simulink model "pos_traj"  (R2017b)
settings: Solver=VariableStepAuto  StartTime=0.0  StopTime=10  RelTol=1e-3
libraries: powerlib_meascontrol x5, mylibrary x2
settings Model: Creator=Kamran  LastModifiedBy=Kamran

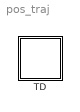
== system pos_traj ==
  TD : Subsystem  mask{h=1e-3, jm=3, am=2, vm=1}

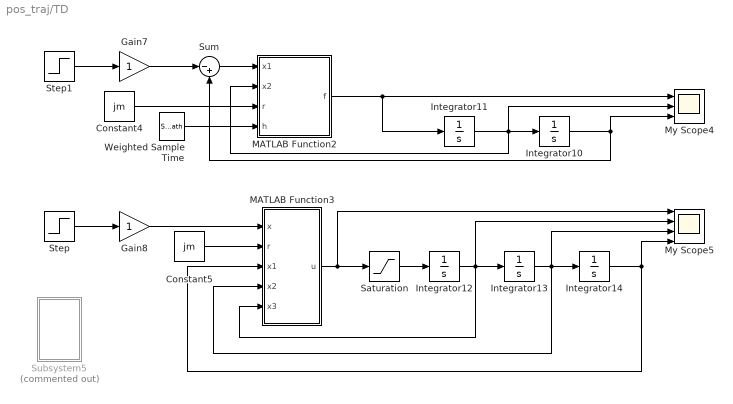
== system pos_traj/TD ==
  Constant4 : Constant  Value=jm
  Constant5 : Constant  Value=jm
  Gain7 : Gain
  Gain8 : Gain
  Integrator10 : Integrator  InitialCondition=0.5  UpperSaturationLimit=vm  LowerSaturationLimit=-vm
  Integrator11 : Integrator  InitialCondition=0.5  LimitOutput=on  UpperSaturationLimit=am  LowerSaturationLimit=-am
  Integrator12 : Integrator  LimitOutput=on  UpperSaturationLimit=sat  LowerSaturationLimit=-sat  ZeroCross=off  mask{sat=am}
  Integrator13 : Integrator  LimitOutput=on  UpperSaturationLimit=sat  LowerSaturationLimit=-sat  ZeroCross=off  mask{sat=vm}
  Integrator14 : Integrator  ZeroCross=off
  MATLAB Function2 : MATLAB Function  TreatAsAtomicUnit=on
  MATLAB Function3 : MATLAB Function  TreatAsAtomicUnit=on
  My Scope4 : Scope  NumInputPorts=3
  My Scope5 : Scope  NumInputPorts=4
  Saturation : Saturate  UpperLimit=sat  LowerLimit=-sat  ZeroCross=off  mask{sat=jm}
  Step : Step  SampleTime=h
  Step1 : Step  Time=0  SampleTime=h
  Subsystem5 : Subsystem  Commented=on
  Sum : Sum  Inputs=|-+
  Weighted Sample Time : SampleTimeMath  TsampMathOp=Ts Only
  wires:
  Saturation/1 -> Integrator12/1
  Integrator12/1 -> My Scope5/2, MATLAB Function3/5(x3), Integrator13/1
  Integrator13/1 -> My Scope5/3, MATLAB Function3/4(x2), Integrator14/1
  Step/1 -> Gain8/1
  Gain8/1 -> MATLAB Function3/1(x)
  MATLAB Function3/1(u) -> Saturation/1, My Scope5/1
  Constant5/1 -> MATLAB Function3/2(r)
  Integrator14/1 -> My Scope5/4, MATLAB Function3/3(x1)
  Integrator10/1 -> Sum/2, My Scope4/3
  Constant4/1 -> MATLAB Function2/3(r)
  Step1/1 -> Gain7/1
  Integrator11/1 -> MATLAB Function2/2(x2), My Scope4/2, Integrator10/1
  Gain7/1 -> Sum/1
  MATLAB Function2/1(f) -> My Scope4/1, Integrator11/1
  Sum/1 -> MATLAB Function2/1(x1)
  Weighted Sample Time/1 -> MATLAB Function2/4(h)

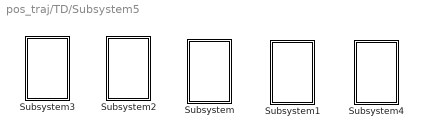
== system pos_traj/TD/Subsystem5 ==
  Subsystem : Subsystem
  Subsystem1 : Subsystem
  Subsystem2 : Subsystem
  Subsystem3 : Subsystem
  Subsystem4 : Subsystem

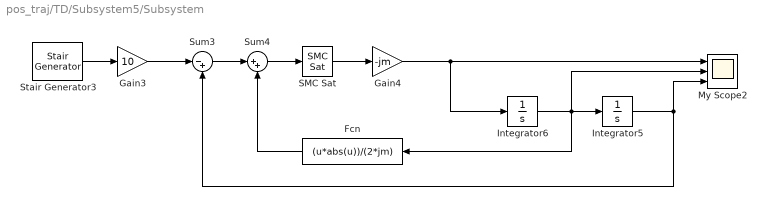
== system pos_traj/TD/Subsystem5/Subsystem ==
  Fcn : Fcn  Expr=(u*abs(u))/(2*jm)
  Gain3 : Gain  Gain=10
  Gain4 : Gain  Gain=-jm
  Integrator5 : Integrator  UpperSaturationLimit=vm  LowerSaturationLimit=-vm
  Integrator6 : Integrator  LimitOutput=on  UpperSaturationLimit=am  LowerSaturationLimit=-am
  My Scope2 : Scope  NumInputPorts=3
  SMC Sat : mylibrary/SMC Sat  psi=eps
      settings: SourceProductName=My Library
  Stair Generator3 : powerlib_meascontrol/Pulse & Signal Generators/Stair Generator  t=[0, 2, 15, 25]  e=[0, 1, 0.1, 0]  Ts=h
      settings: SourceProductName=Simscape Power Systems
  Sum3 : Sum  Inputs=|-+
  Sum4 : Sum  Inputs=|++
  wires:
  Integrator5/1 -> Sum3/2, My Scope2/3
  Sum4/1 -> SMC Sat/1
  Stair Generator3/1 -> Gain3/1
  Gain3/1 -> Sum3/1
  Sum3/1 -> Sum4/1
  Integrator6/1 -> Fcn/1, Integrator5/1, My Scope2/2
  Fcn/1 -> Sum4/2
  Gain4/1 -> Integrator6/1, My Scope2/1
  SMC Sat/1 -> Gain4/1

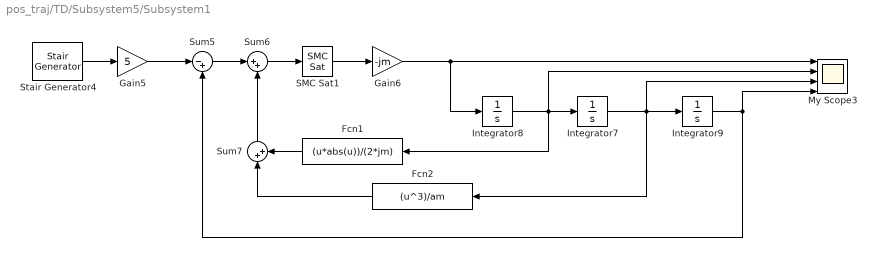
== system pos_traj/TD/Subsystem5/Subsystem1 ==
  Fcn1 : Fcn  Expr=(u*abs(u))/(2*jm)
  Fcn2 : Fcn  Expr=(u^3)/am
  Gain5 : Gain  Gain=5
  Gain6 : Gain  Gain=-jm
  Integrator7 : Integrator  LimitOutput=on  UpperSaturationLimit=vm  LowerSaturationLimit=-vm
  Integrator8 : Integrator  LimitOutput=on  UpperSaturationLimit=am  LowerSaturationLimit=-am
  Integrator9 : Integrator
  My Scope3 : Scope  NumInputPorts=4
  SMC Sat1 : mylibrary/SMC Sat  psi=eps
      settings: SourceProductName=My Library
  Stair Generator4 : powerlib_meascontrol/Pulse & Signal Generators/Stair Generator  t=[0, 2, 15, 25]  e=[0, 1, 0.1, 0]  Ts=h
      settings: SourceProductName=Simscape Power Systems
  Sum5 : Sum  Inputs=|-+
  Sum6 : Sum  Inputs=|++
  Sum7 : Sum  Inputs=|++
  wires:
  Gain6/1 -> My Scope3/1, Integrator8/1
  SMC Sat1/1 -> Gain6/1
  Fcn1/1 -> Sum7/2
  Fcn2/1 -> Sum7/1
  Integrator7/1 -> Fcn2/1, Integrator9/1, My Scope3/3
  Stair Generator4/1 -> Gain5/1
  Sum5/1 -> Sum6/1
  Integrator8/1 -> My Scope3/2, Integrator7/1, Fcn1/1
  Sum6/1 -> SMC Sat1/1
  Integrator9/1 -> Sum5/2, My Scope3/4
  Sum7/1 -> Sum6/2
  Gain5/1 -> Sum5/1

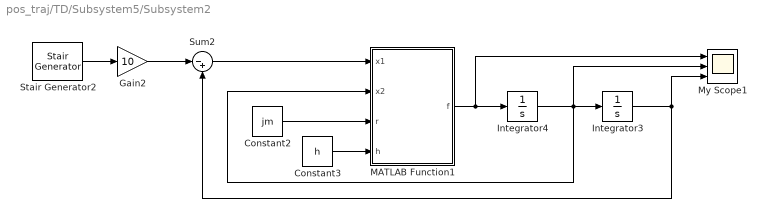
== system pos_traj/TD/Subsystem5/Subsystem2 ==
  Constant2 : Constant  Value=jm
  Constant3 : Constant  Value=h
  Gain2 : Gain  Gain=10
  Integrator3 : Integrator  UpperSaturationLimit=vm  LowerSaturationLimit=-vm
  Integrator4 : Integrator  LimitOutput=on  UpperSaturationLimit=am  LowerSaturationLimit=-am
  MATLAB Function1 : MATLAB Function  TreatAsAtomicUnit=on
  My Scope1 : Scope  NumInputPorts=3
  Stair Generator2 : powerlib_meascontrol/Pulse & Signal Generators/Stair Generator  t=[0, 2, 15, 25]  e=[0, 1, 0.1, 0]  Ts=h
      settings: SourceProductName=Simscape Power Systems
  Sum2 : Sum  Inputs=|-+
  wires:
  Constant3/1 -> MATLAB Function1/4(h)
  Integrator4/1 -> My Scope1/2, MATLAB Function1/2(x2), Integrator3/1
  Sum2/1 -> MATLAB Function1/1(x1)
  Constant2/1 -> MATLAB Function1/3(r)
  Gain2/1 -> Sum2/1
  Integrator3/1 -> My Scope1/3, Sum2/2
  Stair Generator2/1 -> Gain2/1
  MATLAB Function1/1(f) -> My Scope1/1, Integrator4/1

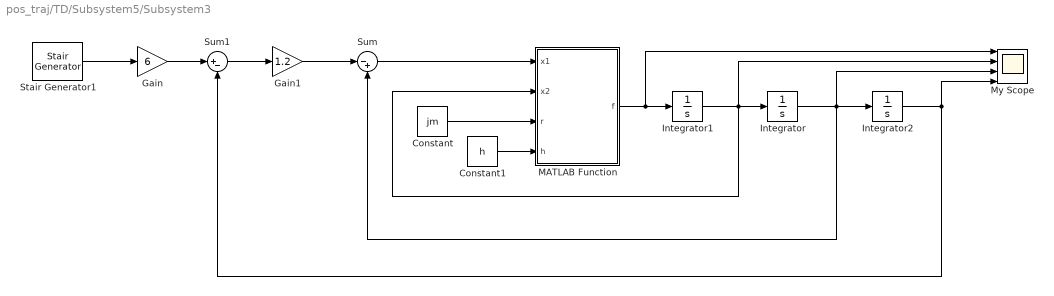
== system pos_traj/TD/Subsystem5/Subsystem3 ==
  Constant : Constant  Value=jm
  Constant1 : Constant  Value=h
  Gain : Gain  Gain=6
  Gain1 : Gain  Gain=1.2
  Integrator : Integrator  LimitOutput=on  UpperSaturationLimit=vm  LowerSaturationLimit=-vm
  Integrator1 : Integrator  LimitOutput=on  UpperSaturationLimit=am  LowerSaturationLimit=-am
  Integrator2 : Integrator
  MATLAB Function : MATLAB Function  TreatAsAtomicUnit=on
  My Scope : Scope  NumInputPorts=4
  Stair Generator1 : powerlib_meascontrol/Pulse & Signal Generators/Stair Generator  t=[0, 2, 15, 25]  e=[0, 1, 0.1, 0]  Ts=h
      settings: SourceProductName=Simscape Power Systems
  Sum : Sum  Inputs=|-+
  Sum1 : Sum  Inputs=|+-
  wires:
  Integrator/1 -> My Scope/3, Sum/2, Integrator2/1
  Constant1/1 -> MATLAB Function/4(h)
  Sum/1 -> MATLAB Function/1(x1)
  Integrator1/1 -> Integrator/1, My Scope/2, MATLAB Function/2(x2)
  Gain1/1 -> Sum/1
  Constant/1 -> MATLAB Function/3(r)
  Gain/1 -> Sum1/1
  Sum1/1 -> Gain1/1
  Stair Generator1/1 -> Gain/1
  Integrator2/1 -> Sum1/2, My Scope/4
  MATLAB Function/1(f) -> My Scope/1, Integrator1/1

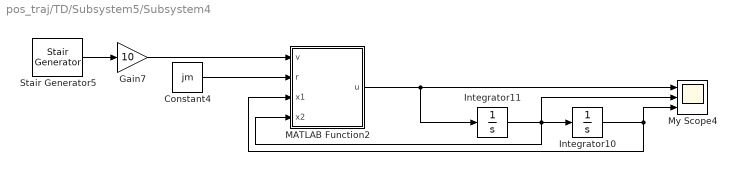
== system pos_traj/TD/Subsystem5/Subsystem4 ==
  Constant4 : Constant  Value=jm
  Gain7 : Gain  Gain=10
  Integrator10 : Integrator  UpperSaturationLimit=vm  LowerSaturationLimit=-vm
  Integrator11 : Integrator  LimitOutput=on  UpperSaturationLimit=am  LowerSaturationLimit=-am
  MATLAB Function2 : MATLAB Function  TreatAsAtomicUnit=on
  My Scope4 : Scope  NumInputPorts=3
  Stair Generator5 : powerlib_meascontrol/Pulse & Signal Generators/Stair Generator  t=[0, 2, 15, 25]  e=[0, 1, 0.1, 0]  Ts=h
      settings: SourceProductName=Simscape Power Systems
  wires:
  Gain7/1 -> MATLAB Function2/1(v)
  MATLAB Function2/1(u) -> My Scope4/1, Integrator11/1
  Integrator11/1 -> MATLAB Function2/4(x2), My Scope4/2, Integrator10/1
  Integrator10/1 -> MATLAB Function2/3(x1), My Scope4/3
  Stair Generator5/1 -> Gain7/1
  Constant4/1 -> MATLAB Function2/2(r)

== matlab function pos_traj/TD/Subsystem5/Subsystem2/MATLAB Function1 ==
  data: x1 input; f output; x2 input; r input; h input
function f = fhan(x1, x2, r, h)

d = r * h^2;
a0 = h * x2;
y = x1 + a0;
a1 = sqrt(d * (d + 8 * abs(y)));
a2 = a0 + sign(y) * (a1 - d) / 2;
sy = (sign(y + d) - sign(y - d)) / 2;
a = (a0 + y - a2) * sy + a2;
sa = (sign(a + d) - sign(a - d)) / 2;
f = -r * (a / d - sign(a)) * sa - r * sign(a);

end

== matlab function pos_traj/TD/Subsystem5/Subsystem4/MATLAB Function2 ==
  data: v input; u output; r input; x1 input; x2 input
function u = fcn(v, r, x1, x2)
    e = v - x1;
    u = r * sat(e - x2 * abs(x2) / (2 * r));
end

function y = sat(s)
    psi = eps;
    if (abs(s) > psi)
        y = sign(s);
    else
        y = s / psi;
    end
end

== matlab function pos_traj/TD/MATLAB Function3 ==
  data: x input; u output; r input; x1 input; x2 input; x3 input
function u  = fcn(x, r, x1, x2, x3)
    s = x1;
    v = x2;
    a = x3;
%     z = v + 0.5 * a * abs(a) / r;
    z = v - a^2/(2*r) * -sat(a);
%     z = s + a^3/(3*r^2) - (a*v)/r * dir(s, v, a);
    u = r * sat(x - z);
end

function d = dir(s, v, a)
    d = 1;
end

function y = sat(s)
    psi = eps;
    if (abs(s) > psi)
        y = sign(s);
    else
        y = s / psi;
    end
end

== matlab function pos_traj/TD/MATLAB Function2 ==
  data: x1 input; x2 input; r input; h input; f output
function f = fhan(x1, x2, r, h)

    d = r * h^2;
    a0 = h * x2;
    y = x1 + a0;
    a1 = sqrt(d * (d + 8 * abs(y)));
    a2 = a0 + sign(y) * (a1 - d) / 2;
    sy = (sign(y + d) - sign(y - d)) / 2;
    a = (a0 + y - a2) * sy + a2;
    sa = (sign(a + d) - sign(a - d)) / 2;
    f = -r * (a / d - sign(a)) * sa - r * sign(a);

end

== matlab function pos_traj/TD/Subsystem5/Subsystem3/MATLAB Function ==
  data: x1 input; f output; x2 input; r input; h input
function f = fhan(x1, x2, r, h)

d = r * h^2;
a0 = h * x2;
y = x1 + a0;
a1 = sqrt(d * (d + 8 * abs(y)));
a2 = a0 + sign(y) * (a1 - d) / 2;
sy = (sign(y + d) - sign(y - d)) / 2;
a = (a0 + y - a2) * sy + a2;
sa = (sign(a + d) - sign(a - d)) / 2;
f = -r * (a / d - sign(a)) * sa - r * sign(a);

end
